simulink model "DriveSystemControl"  (R2023b)
settings: Solver=FixedStepAuto  StartTime=0.0  StopTime=Inf  FixedStep=0.001  RelTol=1e-3
PostLoadFcn:
  | if any(exist('dsrtsu_mdlpostloadfcn', 'file') ~= 0), dsrtsu_mdlpostloadfcn('Execute', bdroot); end
InitFcn:
  | , if any(exist('rtifpga_mdlclblib', 'file') ~= 0), rtifpga_mdlclblib('Init', bdroot); end,
  | , if any(exist('dsmpb_private', 'file') ~= 0), dsmpb_private('dsmpb_mdlclblib', 'Init', bdroot); end,
libraries: dsmpblib x2
(part 7 of 11)

== system DriveSystemControl/Bus Configuration (1) - In/Manipulation/Virya Controller CAN File 08082024/WIP/CANChannel/PDUs/TCU03/sigBPosOvervoltageCutback/Feature Switch ==
  Const_sigBPosOvervoltageCutback Countdown Start Value : Constant  Value=0  OutDataTypeStr=uint32
  Const_sigBPosOvervoltageCutback Feature Switch : Constant  Value=0  OutDataTypeStr=uint32
  _Feature Switch_ : BusCreator  Inputs=2
  Feature Switch : Outport
  wires:
  _Feature Switch_/1 -> Feature Switch/1  "Feature Switch"
  Const_sigBPosOvervoltageCutback Countdown Start Value/1 -> _Feature Switch_/1  "sigBPosOvervoltageCutback Countdown Start Value"
  Const_sigBPosOvervoltageCutback Feature Switch/1 -> _Feature Switch_/2  "sigBPosOvervoltageCutback Feature Switch"

== system DriveSystemControl/Bus Configuration (1) - In/Manipulation/Virya Controller CAN File 08082024/WIP/CANChannel/PDUs/TCU03/sigBPosOvervoltageCutback/ISignal Overwrite Value ==
  Const_sigBPosOvervoltageCutback Overwrite Value : Constant  Value=0  OutDataTypeStr=uint8
  _ISignal Overwrite Value_ : BusCreator  Inputs=1
  ISignal Overwrite Value : Outport
  wires:
  _ISignal Overwrite Value_/1 -> ISignal Overwrite Value/1  "ISignal Overwrite Value"
  Const_sigBPosOvervoltageCutback Overwrite Value/1 -> _ISignal Overwrite Value_/1  "sigBPosOvervoltageCutback Overwrite Value"

== system DriveSystemControl/Bus Configuration (1) - In/Manipulation/Virya Controller CAN File 08082024/WIP/CANChannel/PDUs/TCU03/sigBPosUndervoltageCutback/Feature Switch ==
  Const_sigBPosUndervoltageCutback Countdown Start Value : Constant  Value=0  OutDataTypeStr=uint32
  Const_sigBPosUndervoltageCutback Feature Switch : Constant  Value=0  OutDataTypeStr=uint32
  _Feature Switch_ : BusCreator  Inputs=2
  Feature Switch : Outport
  wires:
  _Feature Switch_/1 -> Feature Switch/1  "Feature Switch"
  Const_sigBPosUndervoltageCutback Countdown Start Value/1 -> _Feature Switch_/1  "sigBPosUndervoltageCutback Countdown Start Value"
  Const_sigBPosUndervoltageCutback Feature Switch/1 -> _Feature Switch_/2  "sigBPosUndervoltageCutback Feature Switch"

== system DriveSystemControl/Bus Configuration (1) - In/Manipulation/Virya Controller CAN File 08082024/WIP/CANChannel/PDUs/TCU03/sigBPosUndervoltageCutback/ISignal Overwrite Value ==
  Const_sigBPosUndervoltageCutback Overwrite Value : Constant  Value=0  OutDataTypeStr=uint8
  _ISignal Overwrite Value_ : BusCreator  Inputs=1
  ISignal Overwrite Value : Outport
  wires:
  _ISignal Overwrite Value_/1 -> ISignal Overwrite Value/1  "ISignal Overwrite Value"
  Const_sigBPosUndervoltageCutback Overwrite Value/1 -> _ISignal Overwrite Value_/1  "sigBPosUndervoltageCutback Overwrite Value"

== system DriveSystemControl/Bus Configuration (1) - In/Manipulation/Virya Controller CAN File 08082024/WIP/CANChannel/PDUs/TCU03/sigBadCalibration/Feature Switch ==
  Const_sigBadCalibration Countdown Start Value : Constant  Value=0  OutDataTypeStr=uint32
  Const_sigBadCalibration Feature Switch : Constant  Value=0  OutDataTypeStr=uint32
  _Feature Switch_ : BusCreator  Inputs=2
  Feature Switch : Outport
  wires:
  _Feature Switch_/1 -> Feature Switch/1  "Feature Switch"
  Const_sigBadCalibration Countdown Start Value/1 -> _Feature Switch_/1  "sigBadCalibration Countdown Start Value"
  Const_sigBadCalibration Feature Switch/1 -> _Feature Switch_/2  "sigBadCalibration Feature Switch"

== system DriveSystemControl/Bus Configuration (1) - In/Manipulation/Virya Controller CAN File 08082024/WIP/CANChannel/PDUs/TCU03/sigBadCalibration/ISignal Overwrite Value ==
  Const_sigBadCalibration Overwrite Value : Constant  Value=0  OutDataTypeStr=uint8
  _ISignal Overwrite Value_ : BusCreator  Inputs=1
  ISignal Overwrite Value : Outport
  wires:
  _ISignal Overwrite Value_/1 -> ISignal Overwrite Value/1  "ISignal Overwrite Value"
  Const_sigBadCalibration Overwrite Value/1 -> _ISignal Overwrite Value_/1  "sigBadCalibration Overwrite Value"

== system DriveSystemControl/Bus Configuration (1) - In/Manipulation/Virya Controller CAN File 08082024/WIP/CANChannel/PDUs/TCU03/sigBrakeWiperHigh/Feature Switch ==
  Const_sigBrakeWiperHigh Countdown Start Value : Constant  Value=0  OutDataTypeStr=uint32
  Const_sigBrakeWiperHigh Feature Switch : Constant  Value=0  OutDataTypeStr=uint32
  _Feature Switch_ : BusCreator  Inputs=2
  Feature Switch : Outport
  wires:
  _Feature Switch_/1 -> Feature Switch/1  "Feature Switch"
  Const_sigBrakeWiperHigh Countdown Start Value/1 -> _Feature Switch_/1  "sigBrakeWiperHigh Countdown Start Value"
  Const_sigBrakeWiperHigh Feature Switch/1 -> _Feature Switch_/2  "sigBrakeWiperHigh Feature Switch"

== system DriveSystemControl/Bus Configuration (1) - In/Manipulation/Virya Controller CAN File 08082024/WIP/CANChannel/PDUs/TCU03/sigBrakeWiperHigh/ISignal Overwrite Value ==
  Const_sigBrakeWiperHigh Overwrite Value : Constant  Value=0  OutDataTypeStr=uint8
  _ISignal Overwrite Value_ : BusCreator  Inputs=1
  ISignal Overwrite Value : Outport
  wires:
  _ISignal Overwrite Value_/1 -> ISignal Overwrite Value/1  "ISignal Overwrite Value"
  Const_sigBrakeWiperHigh Overwrite Value/1 -> _ISignal Overwrite Value_/1  "sigBrakeWiperHigh Overwrite Value"

== system DriveSystemControl/Bus Configuration (1) - In/Manipulation/Virya Controller CAN File 08082024/WIP/CANChannel/PDUs/TCU03/sigBrakeWiperLow/Feature Switch ==
  Const_sigBrakeWiperLow Countdown Start Value : Constant  Value=0  OutDataTypeStr=uint32
  Const_sigBrakeWiperLow Feature Switch : Constant  Value=0  OutDataTypeStr=uint32
  _Feature Switch_ : BusCreator  Inputs=2
  Feature Switch : Outport
  wires:
  _Feature Switch_/1 -> Feature Switch/1  "Feature Switch"
  Const_sigBrakeWiperLow Countdown Start Value/1 -> _Feature Switch_/1  "sigBrakeWiperLow Countdown Start Value"
  Const_sigBrakeWiperLow Feature Switch/1 -> _Feature Switch_/2  "sigBrakeWiperLow Feature Switch"

== system DriveSystemControl/Bus Configuration (1) - In/Manipulation/Virya Controller CAN File 08082024/WIP/CANChannel/PDUs/TCU03/sigBrakeWiperLow/ISignal Overwrite Value ==
  Const_sigBrakeWiperLow Overwrite Value : Constant  Value=0  OutDataTypeStr=uint8
  _ISignal Overwrite Value_ : BusCreator  Inputs=1
  ISignal Overwrite Value : Outport
  wires:
  _ISignal Overwrite Value_/1 -> ISignal Overwrite Value/1  "ISignal Overwrite Value"
  Const_sigBrakeWiperLow Overwrite Value/1 -> _ISignal Overwrite Value_/1  "sigBrakeWiperLow Overwrite Value"

== system DriveSystemControl/Bus Configuration (1) - In/Manipulation/Virya Controller CAN File 08082024/WIP/CANChannel/PDUs/TCU03/sigCoil2DriverOpenShort/Feature Switch ==
  Const_sigCoil2DriverOpenShort Countdown Start Value : Constant  Value=0  OutDataTypeStr=uint32
  Const_sigCoil2DriverOpenShort Feature Switch : Constant  Value=0  OutDataTypeStr=uint32
  _Feature Switch_ : BusCreator  Inputs=2
  Feature Switch : Outport
  wires:
  _Feature Switch_/1 -> Feature Switch/1  "Feature Switch"
  Const_sigCoil2DriverOpenShort Countdown Start Value/1 -> _Feature Switch_/1  "sigCoil2DriverOpenShort Countdown Start Value"
  Const_sigCoil2DriverOpenShort Feature Switch/1 -> _Feature Switch_/2  "sigCoil2DriverOpenShort Feature Switch"

== system DriveSystemControl/Bus Configuration (1) - In/Manipulation/Virya Controller CAN File 08082024/WIP/CANChannel/PDUs/TCU03/sigCoil2DriverOpenShort/ISignal Overwrite Value ==
  Const_sigCoil2DriverOpenShort Overwrite Value : Constant  Value=0  OutDataTypeStr=uint8
  _ISignal Overwrite Value_ : BusCreator  Inputs=1
  ISignal Overwrite Value : Outport
  wires:
  _ISignal Overwrite Value_/1 -> ISignal Overwrite Value/1  "ISignal Overwrite Value"
  Const_sigCoil2DriverOpenShort Overwrite Value/1 -> _ISignal Overwrite Value_/1  "sigCoil2DriverOpenShort Overwrite Value"

== system DriveSystemControl/Bus Configuration (1) - In/Manipulation/Virya Controller CAN File 08082024/WIP/CANChannel/PDUs/TCU03/sigCoil3DriverOpenShort/Feature Switch ==
  Const_sigCoil3DriverOpenShort Countdown Start Value : Constant  Value=0  OutDataTypeStr=uint32
  Const_sigCoil3DriverOpenShort Feature Switch : Constant  Value=0  OutDataTypeStr=uint32
  _Feature Switch_ : BusCreator  Inputs=2
  Feature Switch : Outport
  wires:
  _Feature Switch_/1 -> Feature Switch/1  "Feature Switch"
  Const_sigCoil3DriverOpenShort Countdown Start Value/1 -> _Feature Switch_/1  "sigCoil3DriverOpenShort Countdown Start Value"
  Const_sigCoil3DriverOpenShort Feature Switch/1 -> _Feature Switch_/2  "sigCoil3DriverOpenShort Feature Switch"

== system DriveSystemControl/Bus Configuration (1) - In/Manipulation/Virya Controller CAN File 08082024/WIP/CANChannel/PDUs/TCU03/sigCoil3DriverOpenShort/ISignal Overwrite Value ==
  Const_sigCoil3DriverOpenShort Overwrite Value : Constant  Value=0  OutDataTypeStr=uint8
  _ISignal Overwrite Value_ : BusCreator  Inputs=1
  ISignal Overwrite Value : Outport
  wires:
  _ISignal Overwrite Value_/1 -> ISignal Overwrite Value/1  "ISignal Overwrite Value"
  Const_sigCoil3DriverOpenShort Overwrite Value/1 -> _ISignal Overwrite Value_/1  "sigCoil3DriverOpenShort Overwrite Value"

== system DriveSystemControl/Bus Configuration (1) - In/Manipulation/Virya Controller CAN File 08082024/WIP/CANChannel/PDUs/TCU03/sigCoil4DriverOpenShort/Feature Switch ==
  Const_sigCoil4DriverOpenShort Countdown Start Value : Constant  Value=0  OutDataTypeStr=uint32
  Const_sigCoil4DriverOpenShort Feature Switch : Constant  Value=0  OutDataTypeStr=uint32
  _Feature Switch_ : BusCreator  Inputs=2
  Feature Switch : Outport
  wires:
  _Feature Switch_/1 -> Feature Switch/1  "Feature Switch"
  Const_sigCoil4DriverOpenShort Countdown Start Value/1 -> _Feature Switch_/1  "sigCoil4DriverOpenShort Countdown Start Value"
  Const_sigCoil4DriverOpenShort Feature Switch/1 -> _Feature Switch_/2  "sigCoil4DriverOpenShort Feature Switch"

== system DriveSystemControl/Bus Configuration (1) - In/Manipulation/Virya Controller CAN File 08082024/WIP/CANChannel/PDUs/TCU03/sigCoil4DriverOpenShort/ISignal Overwrite Value ==
  Const_sigCoil4DriverOpenShort Overwrite Value : Constant  Value=0  OutDataTypeStr=uint8
  _ISignal Overwrite Value_ : BusCreator  Inputs=1
  ISignal Overwrite Value : Outport
  wires:
  _ISignal Overwrite Value_/1 -> ISignal Overwrite Value/1  "ISignal Overwrite Value"
  Const_sigCoil4DriverOpenShort Overwrite Value/1 -> _ISignal Overwrite Value_/1  "sigCoil4DriverOpenShort Overwrite Value"

== system DriveSystemControl/Bus Configuration (1) - In/Manipulation/Virya Controller CAN File 08082024/WIP/CANChannel/PDUs/TCU03/sigControllerCommonFault/Feature Switch ==
  Const_sigControllerCommonFault Countdown Start Value : Constant  Value=0  OutDataTypeStr=uint32
  Const_sigControllerCommonFault Feature Switch : Constant  Value=0  OutDataTypeStr=uint32
  _Feature Switch_ : BusCreator  Inputs=2
  Feature Switch : Outport
  wires:
  _Feature Switch_/1 -> Feature Switch/1  "Feature Switch"
  Const_sigControllerCommonFault Countdown Start Value/1 -> _Feature Switch_/1  "sigControllerCommonFault Countdown Start Value"
  Const_sigControllerCommonFault Feature Switch/1 -> _Feature Switch_/2  "sigControllerCommonFault Feature Switch"

== system DriveSystemControl/Bus Configuration (1) - In/Manipulation/Virya Controller CAN File 08082024/WIP/CANChannel/PDUs/TCU03/sigControllerCommonFault/ISignal Overwrite Value ==
  Const_sigControllerCommonFault Overwrite Value : Constant  Value=0  OutDataTypeStr=uint8
  _ISignal Overwrite Value_ : BusCreator  Inputs=1
  ISignal Overwrite Value : Outport
  wires:
  _ISignal Overwrite Value_/1 -> ISignal Overwrite Value/1  "ISignal Overwrite Value"
  Const_sigControllerCommonFault Overwrite Value/1 -> _ISignal Overwrite Value_/1  "sigControllerCommonFault Overwrite Value"

== system DriveSystemControl/Bus Configuration (1) - In/Manipulation/Virya Controller CAN File 08082024/WIP/CANChannel/PDUs/TCU03/sigControllerOverCurrent/Feature Switch ==
  Const_sigControllerOverCurrent Countdown Start Value : Constant  Value=0  OutDataTypeStr=uint32
  Const_sigControllerOverCurrent Feature Switch : Constant  Value=0  OutDataTypeStr=uint32
  _Feature Switch_ : BusCreator  Inputs=2
  Feature Switch : Outport
  wires:
  _Feature Switch_/1 -> Feature Switch/1  "Feature Switch"
  Const_sigControllerOverCurrent Countdown Start Value/1 -> _Feature Switch_/1  "sigControllerOverCurrent Countdown Start Value"
  Const_sigControllerOverCurrent Feature Switch/1 -> _Feature Switch_/2  "sigControllerOverCurrent Feature Switch"

== system DriveSystemControl/Bus Configuration (1) - In/Manipulation/Virya Controller CAN File 08082024/WIP/CANChannel/PDUs/TCU03/sigControllerOverCurrent/ISignal Overwrite Value ==
  Const_sigControllerOverCurrent Overwrite Value : Constant  Value=0  OutDataTypeStr=uint8
  _ISignal Overwrite Value_ : BusCreator  Inputs=1
  ISignal Overwrite Value : Outport
  wires:
  _ISignal Overwrite Value_/1 -> ISignal Overwrite Value/1  "ISignal Overwrite Value"
  Const_sigControllerOverCurrent Overwrite Value/1 -> _ISignal Overwrite Value_/1  "sigControllerOverCurrent Overwrite Value"

== system DriveSystemControl/Bus Configuration (1) - In/Manipulation/Virya Controller CAN File 08082024/WIP/CANChannel/PDUs/TCU03/sigControllerOvertempCutback/Feature Switch ==
  Const_sigControllerOvertempCutback Countdown Start Value : Constant  Value=0  OutDataTypeStr=uint32
  Const_sigControllerOvertempCutback Feature Switch : Constant  Value=0  OutDataTypeStr=uint32
  _Feature Switch_ : BusCreator  Inputs=2
  Feature Switch : Outport
  wires:
  _Feature Switch_/1 -> Feature Switch/1  "Feature Switch"
  Const_sigControllerOvertempCutback Countdown Start Value/1 -> _Feature Switch_/1  "sigControllerOvertempCutback Countdown Start Value"
  Const_sigControllerOvertempCutback Feature Switch/1 -> _Feature Switch_/2  "sigControllerOvertempCutback Feature Switch"

== system DriveSystemControl/Bus Configuration (1) - In/Manipulation/Virya Controller CAN File 08082024/WIP/CANChannel/PDUs/TCU03/sigControllerOvertempCutback/ISignal Overwrite Value ==
  Const_sigControllerOvertempCutback Overwrite Value : Constant  Value=0  OutDataTypeStr=uint8
  _ISignal Overwrite Value_ : BusCreator  Inputs=1
  ISignal Overwrite Value : Outport
  wires:
  _ISignal Overwrite Value_/1 -> ISignal Overwrite Value/1  "ISignal Overwrite Value"
  Const_sigControllerOvertempCutback Overwrite Value/1 -> _ISignal Overwrite Value_/1  "sigControllerOvertempCutback Overwrite Value"

== system DriveSystemControl/Bus Configuration (1) - In/Manipulation/Virya Controller CAN File 08082024/WIP/CANChannel/PDUs/TCU03/sigControllerSevereOvertemp/Feature Switch ==
  Const_sigControllerSevereOvertemp Countdown Start Value : Constant  Value=0  OutDataTypeStr=uint32
  Const_sigControllerSevereOvertemp Feature Switch : Constant  Value=0  OutDataTypeStr=uint32
  _Feature Switch_ : BusCreator  Inputs=2
  Feature Switch : Outport
  wires:
  _Feature Switch_/1 -> Feature Switch/1  "Feature Switch"
  Const_sigControllerSevereOvertemp Countdown Start Value/1 -> _Feature Switch_/1  "sigControllerSevereOvertemp Countdown Start Value"
  Const_sigControllerSevereOvertemp Feature Switch/1 -> _Feature Switch_/2  "sigControllerSevereOvertemp Feature Switch"

== system DriveSystemControl/Bus Configuration (1) - In/Manipulation/Virya Controller CAN File 08082024/WIP/CANChannel/PDUs/TCU03/sigControllerSevereOvertemp/ISignal Overwrite Value ==
  Const_sigControllerSevereOvertemp Overwrite Value : Constant  Value=0  OutDataTypeStr=uint8
  _ISignal Overwrite Value_ : BusCreator  Inputs=1
  ISignal Overwrite Value : Outport
  wires:
  _ISignal Overwrite Value_/1 -> ISignal Overwrite Value/1  "ISignal Overwrite Value"
  Const_sigControllerSevereOvertemp Overwrite Value/1 -> _ISignal Overwrite Value_/1  "sigControllerSevereOvertemp Overwrite Value"

== system DriveSystemControl/Bus Configuration (1) - In/Manipulation/Virya Controller CAN File 08082024/WIP/CANChannel/PDUs/TCU03/sigControllerSevereUndertemp/Feature Switch ==
  Const_sigControllerSevereUndertemp Countdown Start Value : Constant  Value=0  OutDataTypeStr=uint32
  Const_sigControllerSevereUndertemp Feature Switch : Constant  Value=0  OutDataTypeStr=uint32
  _Feature Switch_ : BusCreator  Inputs=2
  Feature Switch : Outport
  wires:
  _Feature Switch_/1 -> Feature Switch/1  "Feature Switch"
  Const_sigControllerSevereUndertemp Countdown Start Value/1 -> _Feature Switch_/1  "sigControllerSevereUndertemp Countdown Start Value"
  Const_sigControllerSevereUndertemp Feature Switch/1 -> _Feature Switch_/2  "sigControllerSevereUndertemp Feature Switch"

== system DriveSystemControl/Bus Configuration (1) - In/Manipulation/Virya Controller CAN File 08082024/WIP/CANChannel/PDUs/TCU03/sigControllerSevereUndertemp/ISignal Overwrite Value ==
  Const_sigControllerSevereUndertemp Overwrite Value : Constant  Value=0  OutDataTypeStr=uint8
  _ISignal Overwrite Value_ : BusCreator  Inputs=1
  ISignal Overwrite Value : Outport
  wires:
  _ISignal Overwrite Value_/1 -> ISignal Overwrite Value/1  "ISignal Overwrite Value"
  Const_sigControllerSevereUndertemp Overwrite Value/1 -> _ISignal Overwrite Value_/1  "sigControllerSevereUndertemp Overwrite Value"

== system DriveSystemControl/Bus Configuration (1) - In/Manipulation/Virya Controller CAN File 08082024/WIP/CANChannel/PDUs/TCU03/sigCurrentSensorFault/Feature Switch ==
  Const_sigCurrentSensorFault Countdown Start Value : Constant  Value=0  OutDataTypeStr=uint32
  Const_sigCurrentSensorFault Feature Switch : Constant  Value=0  OutDataTypeStr=uint32
  _Feature Switch_ : BusCreator  Inputs=2
  Feature Switch : Outport
  wires:
  _Feature Switch_/1 -> Feature Switch/1  "Feature Switch"
  Const_sigCurrentSensorFault Countdown Start Value/1 -> _Feature Switch_/1  "sigCurrentSensorFault Countdown Start Value"
  Const_sigCurrentSensorFault Feature Switch/1 -> _Feature Switch_/2  "sigCurrentSensorFault Feature Switch"

== system DriveSystemControl/Bus Configuration (1) - In/Manipulation/Virya Controller CAN File 08082024/WIP/CANChannel/PDUs/TCU03/sigCurrentSensorFault/ISignal Overwrite Value ==
  Const_sigCurrentSensorFault Overwrite Value : Constant  Value=0  OutDataTypeStr=uint8
  _ISignal Overwrite Value_ : BusCreator  Inputs=1
  ISignal Overwrite Value : Outport
  wires:
  _ISignal Overwrite Value_/1 -> ISignal Overwrite Value/1  "ISignal Overwrite Value"
  Const_sigCurrentSensorFault Overwrite Value/1 -> _ISignal Overwrite Value_/1  "sigCurrentSensorFault Overwrite Value"

== system DriveSystemControl/Bus Configuration (1) - In/Manipulation/Virya Controller CAN File 08082024/WIP/CANChannel/PDUs/TCU03/sigEEPROMFailure/Feature Switch ==
  Const_sigEEPROMFailure Countdown Start Value : Constant  Value=0  OutDataTypeStr=uint32
  Const_sigEEPROMFailure Feature Switch : Constant  Value=0  OutDataTypeStr=uint32
  _Feature Switch_ : BusCreator  Inputs=2
  Feature Switch : Outport
  wires:
  _Feature Switch_/1 -> Feature Switch/1  "Feature Switch"
  Const_sigEEPROMFailure Countdown Start Value/1 -> _Feature Switch_/1  "sigEEPROMFailure Countdown Start Value"
  Const_sigEEPROMFailure Feature Switch/1 -> _Feature Switch_/2  "sigEEPROMFailure Feature Switch"

== system DriveSystemControl/Bus Configuration (1) - In/Manipulation/Virya Controller CAN File 08082024/WIP/CANChannel/PDUs/TCU03/sigEEPROMFailure/ISignal Overwrite Value ==
  Const_sigEEPROMFailure Overwrite Value : Constant  Value=0  OutDataTypeStr=uint8
  _ISignal Overwrite Value_ : BusCreator  Inputs=1
  ISignal Overwrite Value : Outport
  wires:
  _ISignal Overwrite Value_/1 -> ISignal Overwrite Value/1  "ISignal Overwrite Value"
  Const_sigEEPROMFailure Overwrite Value/1 -> _ISignal Overwrite Value_/1  "sigEEPROMFailure Overwrite Value"

== system DriveSystemControl/Bus Configuration (1) - In/Manipulation/Virya Controller CAN File 08082024/WIP/CANChannel/PDUs/TCU03/sigHighPedalDisable/Feature Switch ==
  Const_sigHighPedalDisable Countdown Start Value : Constant  Value=0  OutDataTypeStr=uint32
  Const_sigHighPedalDisable Feature Switch : Constant  Value=0  OutDataTypeStr=uint32
  _Feature Switch_ : BusCreator  Inputs=2
  Feature Switch : Outport
  wires:
  _Feature Switch_/1 -> Feature Switch/1  "Feature Switch"
  Const_sigHighPedalDisable Countdown Start Value/1 -> _Feature Switch_/1  "sigHighPedalDisable Countdown Start Value"
  Const_sigHighPedalDisable Feature Switch/1 -> _Feature Switch_/2  "sigHighPedalDisable Feature Switch"

== system DriveSystemControl/Bus Configuration (1) - In/Manipulation/Virya Controller CAN File 08082024/WIP/CANChannel/PDUs/TCU03/sigHighPedalDisable/ISignal Overwrite Value ==
  Const_sigHighPedalDisable Overwrite Value : Constant  Value=0  OutDataTypeStr=uint8
  _ISignal Overwrite Value_ : BusCreator  Inputs=1
  ISignal Overwrite Value : Outport
  wires:
  _ISignal Overwrite Value_/1 -> ISignal Overwrite Value/1  "ISignal Overwrite Value"
  Const_sigHighPedalDisable Overwrite Value/1 -> _ISignal Overwrite Value_/1  "sigHighPedalDisable Overwrite Value"

== system DriveSystemControl/Bus Configuration (1) - In/Manipulation/Virya Controller CAN File 08082024/WIP/CANChannel/PDUs/TCU03/sigInsulationResistanceLow/Feature Switch ==
  Const_sigInsulationResistanceLow Countdown Start Value : Constant  Value=0  OutDataTypeStr=uint32
  Const_sigInsulationResistanceLow Feature Switch : Constant  Value=0  OutDataTypeStr=uint32
  _Feature Switch_ : BusCreator  Inputs=2
  Feature Switch : Outport
  wires:
  _Feature Switch_/1 -> Feature Switch/1  "Feature Switch"
  Const_sigInsulationResistanceLow Countdown Start Value/1 -> _Feature Switch_/1  "sigInsulationResistanceLow Countdown Start Value"
  Const_sigInsulationResistanceLow Feature Switch/1 -> _Feature Switch_/2  "sigInsulationResistanceLow Feature Switch"

== system DriveSystemControl/Bus Configuration (1) - In/Manipulation/Virya Controller CAN File 08082024/WIP/CANChannel/PDUs/TCU03/sigInsulationResistanceLow/ISignal Overwrite Value ==
  Const_sigInsulationResistanceLow Overwrite Value : Constant  Value=0  OutDataTypeStr=uint8
  _ISignal Overwrite Value_ : BusCreator  Inputs=1
  ISignal Overwrite Value : Outport
  wires:
  _ISignal Overwrite Value_/1 -> ISignal Overwrite Value/1  "ISignal Overwrite Value"
  Const_sigInsulationResistanceLow Overwrite Value/1 -> _ISignal Overwrite Value_/1  "sigInsulationResistanceLow Overwrite Value"

== system DriveSystemControl/Bus Configuration (1) - In/Manipulation/Virya Controller CAN File 08082024/WIP/CANChannel/PDUs/TCU03/sigMainContactorWelded/Feature Switch ==
  Const_sigMainContactorWelded Countdown Start Value : Constant  Value=0  OutDataTypeStr=uint32
  Const_sigMainContactorWelded Feature Switch : Constant  Value=0  OutDataTypeStr=uint32
  _Feature Switch_ : BusCreator  Inputs=2
  Feature Switch : Outport
  wires:
  _Feature Switch_/1 -> Feature Switch/1  "Feature Switch"
  Const_sigMainContactorWelded Countdown Start Value/1 -> _Feature Switch_/1  "sigMainContactorWelded Countdown Start Value"
  Const_sigMainContactorWelded Feature Switch/1 -> _Feature Switch_/2  "sigMainContactorWelded Feature Switch"

== system DriveSystemControl/Bus Configuration (1) - In/Manipulation/Virya Controller CAN File 08082024/WIP/CANChannel/PDUs/TCU03/sigMainContactorWelded/ISignal Overwrite Value ==
  Const_sigMainContactorWelded Overwrite Value : Constant  Value=0  OutDataTypeStr=uint8
  _ISignal Overwrite Value_ : BusCreator  Inputs=1
  ISignal Overwrite Value : Outport
  wires:
  _ISignal Overwrite Value_/1 -> ISignal Overwrite Value/1  "ISignal Overwrite Value"
  Const_sigMainContactorWelded Overwrite Value/1 -> _ISignal Overwrite Value_/1  "sigMainContactorWelded Overwrite Value"

== system DriveSystemControl/Bus Configuration (1) - In/Manipulation/Virya Controller CAN File 08082024/WIP/CANChannel/PDUs/TCU03/sigMainContactordidnotClose/Feature Switch ==
  Const_sigMainContactordidnotClose Countdown Start Value : Constant  Value=0  OutDataTypeStr=uint32
  Const_sigMainContactordidnotClose Feature Switch : Constant  Value=0  OutDataTypeStr=uint32
  _Feature Switch_ : BusCreator  Inputs=2
  Feature Switch : Outport
  wires:
  _Feature Switch_/1 -> Feature Switch/1  "Feature Switch"
  Const_sigMainContactordidnotClose Countdown Start Value/1 -> _Feature Switch_/1  "sigMainContactordidnotClose Countdown Start Value"
  Const_sigMainContactordidnotClose Feature Switch/1 -> _Feature Switch_/2  "sigMainContactordidnotClose Feature Switch"

== system DriveSystemControl/Bus Configuration (1) - In/Manipulation/Virya Controller CAN File 08082024/WIP/CANChannel/PDUs/TCU03/sigMainContactordidnotClose/ISignal Overwrite Value ==
  Const_sigMainContactordidnotClose Overwrite Value : Constant  Value=0  OutDataTypeStr=uint8
  _ISignal Overwrite Value_ : BusCreator  Inputs=1
  ISignal Overwrite Value : Outport
  wires:
  _ISignal Overwrite Value_/1 -> ISignal Overwrite Value/1  "ISignal Overwrite Value"
  Const_sigMainContactordidnotClose Overwrite Value/1 -> _ISignal Overwrite Value_/1  "sigMainContactordidnotClose Overwrite Value"

== system DriveSystemControl/Bus Configuration (1) - In/Manipulation/Virya Controller CAN File 08082024/WIP/CANChannel/PDUs/TCU03/sigMainOpenShort/Feature Switch ==
  Const_sigMainOpenShort Countdown Start Value : Constant  Value=0  OutDataTypeStr=uint32
  Const_sigMainOpenShort Feature Switch : Constant  Value=0  OutDataTypeStr=uint32
  _Feature Switch_ : BusCreator  Inputs=2
  Feature Switch : Outport
  wires:
  _Feature Switch_/1 -> Feature Switch/1  "Feature Switch"
  Const_sigMainOpenShort Countdown Start Value/1 -> _Feature Switch_/1  "sigMainOpenShort Countdown Start Value"
  Const_sigMainOpenShort Feature Switch/1 -> _Feature Switch_/2  "sigMainOpenShort Feature Switch"

== system DriveSystemControl/Bus Configuration (1) - In/Manipulation/Virya Controller CAN File 08082024/WIP/CANChannel/PDUs/TCU03/sigMainOpenShort/ISignal Overwrite Value ==
  Const_sigMainOpenShort Overwrite Value : Constant  Value=0  OutDataTypeStr=uint8
  _ISignal Overwrite Value_ : BusCreator  Inputs=1
  ISignal Overwrite Value : Outport
  wires:
  _ISignal Overwrite Value_/1 -> ISignal Overwrite Value/1  "ISignal Overwrite Value"
  Const_sigMainOpenShort Overwrite Value/1 -> _ISignal Overwrite Value_/1  "sigMainOpenShort Overwrite Value"

== system DriveSystemControl/Bus Configuration (1) - In/Manipulation/Virya Controller CAN File 08082024/WIP/CANChannel/PDUs/TCU03/sigMotorCharacterization/Feature Switch ==
  Const_sigMotorCharacterization Countdown Start Value : Constant  Value=0  OutDataTypeStr=uint32
  Const_sigMotorCharacterization Feature Switch : Constant  Value=0  OutDataTypeStr=uint32
  _Feature Switch_ : BusCreator  Inputs=2
  Feature Switch : Outport
  wires:
  _Feature Switch_/1 -> Feature Switch/1  "Feature Switch"
  Const_sigMotorCharacterization Countdown Start Value/1 -> _Feature Switch_/1  "sigMotorCharacterization Countdown Start Value"
  Const_sigMotorCharacterization Feature Switch/1 -> _Feature Switch_/2  "sigMotorCharacterization Feature Switch"

== system DriveSystemControl/Bus Configuration (1) - In/Manipulation/Virya Controller CAN File 08082024/WIP/CANChannel/PDUs/TCU03/sigMotorCharacterization/ISignal Overwrite Value ==
  Const_sigMotorCharacterization Overwrite Value : Constant  Value=0  OutDataTypeStr=uint8
  _ISignal Overwrite Value_ : BusCreator  Inputs=1
  ISignal Overwrite Value : Outport
  wires:
  _ISignal Overwrite Value_/1 -> ISignal Overwrite Value/1  "ISignal Overwrite Value"
  Const_sigMotorCharacterization Overwrite Value/1 -> _ISignal Overwrite Value_/1  "sigMotorCharacterization Overwrite Value"

== system DriveSystemControl/Bus Configuration (1) - In/Manipulation/Virya Controller CAN File 08082024/WIP/CANChannel/PDUs/TCU03/sigMotorPhaseOpen/Feature Switch ==
  Const_sigMotorPhaseOpen Countdown Start Value : Constant  Value=0  OutDataTypeStr=uint32
  Const_sigMotorPhaseOpen Feature Switch : Constant  Value=0  OutDataTypeStr=uint32
  _Feature Switch_ : BusCreator  Inputs=2
  Feature Switch : Outport
  wires:
  _Feature Switch_/1 -> Feature Switch/1  "Feature Switch"
  Const_sigMotorPhaseOpen Countdown Start Value/1 -> _Feature Switch_/1  "sigMotorPhaseOpen Countdown Start Value"
  Const_sigMotorPhaseOpen Feature Switch/1 -> _Feature Switch_/2  "sigMotorPhaseOpen Feature Switch"

== system DriveSystemControl/Bus Configuration (1) - In/Manipulation/Virya Controller CAN File 08082024/WIP/CANChannel/PDUs/TCU03/sigMotorPhaseOpen/ISignal Overwrite Value ==
  Const_sigMotorPhaseOpen Overwrite Value : Constant  Value=0  OutDataTypeStr=uint8
  _ISignal Overwrite Value_ : BusCreator  Inputs=1
  ISignal Overwrite Value : Outport
  wires:
  _ISignal Overwrite Value_/1 -> ISignal Overwrite Value/1  "ISignal Overwrite Value"
  Const_sigMotorPhaseOpen Overwrite Value/1 -> _ISignal Overwrite Value_/1  "sigMotorPhaseOpen Overwrite Value"

== system DriveSystemControl/Bus Configuration (1) - In/Manipulation/Virya Controller CAN File 08082024/WIP/CANChannel/PDUs/TCU03/sigMotorTempHotCutback/Feature Switch ==
  Const_sigMotorTempHotCutback Countdown Start Value : Constant  Value=0  OutDataTypeStr=uint32
  Const_sigMotorTempHotCutback Feature Switch : Constant  Value=0  OutDataTypeStr=uint32
  _Feature Switch_ : BusCreator  Inputs=2
  Feature Switch : Outport
  wires:
  _Feature Switch_/1 -> Feature Switch/1  "Feature Switch"
  Const_sigMotorTempHotCutback Countdown Start Value/1 -> _Feature Switch_/1  "sigMotorTempHotCutback Countdown Start Value"
  Const_sigMotorTempHotCutback Feature Switch/1 -> _Feature Switch_/2  "sigMotorTempHotCutback Feature Switch"

== system DriveSystemControl/Bus Configuration (1) - In/Manipulation/Virya Controller CAN File 08082024/WIP/CANChannel/PDUs/TCU03/sigMotorTempHotCutback/ISignal Overwrite Value ==
  Const_sigMotorTempHotCutback Overwrite Value : Constant  Value=0  OutDataTypeStr=uint8
  _ISignal Overwrite Value_ : BusCreator  Inputs=1
  ISignal Overwrite Value : Outport
  wires:
  _ISignal Overwrite Value_/1 -> ISignal Overwrite Value/1  "ISignal Overwrite Value"
  Const_sigMotorTempHotCutback Overwrite Value/1 -> _ISignal Overwrite Value_/1  "sigMotorTempHotCutback Overwrite Value"

== system DriveSystemControl/Bus Configuration (1) - In/Manipulation/Virya Controller CAN File 08082024/WIP/CANChannel/PDUs/TCU03/sigMotorTempSensorFault/Feature Switch ==
  Const_sigMotorTempSensorFault Countdown Start Value : Constant  Value=0  OutDataTypeStr=uint32
  Const_sigMotorTempSensorFault Feature Switch : Constant  Value=0  OutDataTypeStr=uint32
  _Feature Switch_ : BusCreator  Inputs=2
  Feature Switch : Outport
  wires:
  _Feature Switch_/1 -> Feature Switch/1  "Feature Switch"
  Const_sigMotorTempSensorFault Countdown Start Value/1 -> _Feature Switch_/1  "sigMotorTempSensorFault Countdown Start Value"
  Const_sigMotorTempSensorFault Feature Switch/1 -> _Feature Switch_/2  "sigMotorTempSensorFault Feature Switch"

== system DriveSystemControl/Bus Configuration (1) - In/Manipulation/Virya Controller CAN File 08082024/WIP/CANChannel/PDUs/TCU03/sigMotorTempSensorFault/ISignal Overwrite Value ==
  Const_sigMotorTempSensorFault Overwrite Value : Constant  Value=0  OutDataTypeStr=uint8
  _ISignal Overwrite Value_ : BusCreator  Inputs=1
  ISignal Overwrite Value : Outport
  wires:
  _ISignal Overwrite Value_/1 -> ISignal Overwrite Value/1  "ISignal Overwrite Value"
  Const_sigMotorTempSensorFault Overwrite Value/1 -> _ISignal Overwrite Value_/1  "sigMotorTempSensorFault Overwrite Value"

== system DriveSystemControl/Bus Configuration (1) - In/Manipulation/Virya Controller CAN File 08082024/WIP/CANChannel/PDUs/TCU03/sigOEM_BatterySTOPSignal/Feature Switch ==
  Const_sigOEM_BatterySTOPSignal Countdown Start Value : Constant  Value=0  OutDataTypeStr=uint32
  Const_sigOEM_BatterySTOPSignal Feature Switch : Constant  Value=0  OutDataTypeStr=uint32
  _Feature Switch_ : BusCreator  Inputs=2
  Feature Switch : Outport
  wires:
  _Feature Switch_/1 -> Feature Switch/1  "Feature Switch"
  Const_sigOEM_BatterySTOPSignal Countdown Start Value/1 -> _Feature Switch_/1  "sigOEM_BatterySTOPSignal Countdown Start Value"
  Const_sigOEM_BatterySTOPSignal Feature Switch/1 -> _Feature Switch_/2  "sigOEM_BatterySTOPSignal Feature Switch"

== system DriveSystemControl/Bus Configuration (1) - In/Manipulation/Virya Controller CAN File 08082024/WIP/CANChannel/PDUs/TCU03/sigOEM_BatterySTOPSignal/ISignal Overwrite Value ==
  Const_sigOEM_BatterySTOPSignal Overwrite Value : Constant  Value=0  OutDataTypeStr=uint8
  _ISignal Overwrite Value_ : BusCreator  Inputs=1
  ISignal Overwrite Value : Outport
  wires:
  _ISignal Overwrite Value_/1 -> ISignal Overwrite Value/1  "ISignal Overwrite Value"
  Const_sigOEM_BatterySTOPSignal Overwrite Value/1 -> _ISignal Overwrite Value_/1  "sigOEM_BatterySTOPSignal Overwrite Value"

== system DriveSystemControl/Bus Configuration (1) - In/Manipulation/Virya Controller CAN File 08082024/WIP/CANChannel/PDUs/TCU03/sigOEM_NoBatteryCAN/Feature Switch ==
  Const_sigOEM_NoBatteryCAN Countdown Start Value : Constant  Value=0  OutDataTypeStr=uint32
  Const_sigOEM_NoBatteryCAN Feature Switch : Constant  Value=0  OutDataTypeStr=uint32
  _Feature Switch_ : BusCreator  Inputs=2
  Feature Switch : Outport
  wires:
  _Feature Switch_/1 -> Feature Switch/1  "Feature Switch"
  Const_sigOEM_NoBatteryCAN Countdown Start Value/1 -> _Feature Switch_/1  "sigOEM_NoBatteryCAN Countdown Start Value"
  Const_sigOEM_NoBatteryCAN Feature Switch/1 -> _Feature Switch_/2  "sigOEM_NoBatteryCAN Feature Switch"

== system DriveSystemControl/Bus Configuration (1) - In/Manipulation/Virya Controller CAN File 08082024/WIP/CANChannel/PDUs/TCU03/sigOEM_NoBatteryCAN/ISignal Overwrite Value ==
  Const_sigOEM_NoBatteryCAN Overwrite Value : Constant  Value=0  OutDataTypeStr=uint8
  _ISignal Overwrite Value_ : BusCreator  Inputs=1
  ISignal Overwrite Value : Outport
  wires:
  _ISignal Overwrite Value_/1 -> ISignal Overwrite Value/1  "ISignal Overwrite Value"
  Const_sigOEM_NoBatteryCAN Overwrite Value/1 -> _ISignal Overwrite Value_/1  "sigOEM_NoBatteryCAN Overwrite Value"

== system DriveSystemControl/Bus Configuration (1) - In/Manipulation/Virya Controller CAN File 08082024/WIP/CANChannel/PDUs/TCU03/sigOSGeneral/Feature Switch ==
  Const_sigOSGeneral Countdown Start Value : Constant  Value=0  OutDataTypeStr=uint32
  Const_sigOSGeneral Feature Switch : Constant  Value=0  OutDataTypeStr=uint32
  _Feature Switch_ : BusCreator  Inputs=2
  Feature Switch : Outport
  wires:
  _Feature Switch_/1 -> Feature Switch/1  "Feature Switch"
  Const_sigOSGeneral Countdown Start Value/1 -> _Feature Switch_/1  "sigOSGeneral Countdown Start Value"
  Const_sigOSGeneral Feature Switch/1 -> _Feature Switch_/2  "sigOSGeneral Feature Switch"

== system DriveSystemControl/Bus Configuration (1) - In/Manipulation/Virya Controller CAN File 08082024/WIP/CANChannel/PDUs/TCU03/sigOSGeneral/ISignal Overwrite Value ==
  Const_sigOSGeneral Overwrite Value : Constant  Value=0  OutDataTypeStr=uint8
  _ISignal Overwrite Value_ : BusCreator  Inputs=1
  ISignal Overwrite Value : Outport
  wires:
  _ISignal Overwrite Value_/1 -> ISignal Overwrite Value/1  "ISignal Overwrite Value"
  Const_sigOSGeneral Overwrite Value/1 -> _ISignal Overwrite Value_/1  "sigOSGeneral Overwrite Value"

== system DriveSystemControl/Bus Configuration (1) - In/Manipulation/Virya Controller CAN File 08082024/WIP/CANChannel/PDUs/TCU03/sigPMACCommissioningNeeded/Feature Switch ==
  Const_sigPMACCommissioningNeeded Countdown Start Value : Constant  Value=0  OutDataTypeStr=uint32
  Const_sigPMACCommissioningNeeded Feature Switch : Constant  Value=0  OutDataTypeStr=uint32
  _Feature Switch_ : BusCreator  Inputs=2
  Feature Switch : Outport
  wires:
  _Feature Switch_/1 -> Feature Switch/1  "Feature Switch"
  Const_sigPMACCommissioningNeeded Countdown Start Value/1 -> _Feature Switch_/1  "sigPMACCommissioningNeeded Countdown Start Value"
  Const_sigPMACCommissioningNeeded Feature Switch/1 -> _Feature Switch_/2  "sigPMACCommissioningNeeded Feature Switch"

== system DriveSystemControl/Bus Configuration (1) - In/Manipulation/Virya Controller CAN File 08082024/WIP/CANChannel/PDUs/TCU03/sigPMACCommissioningNeeded/ISignal Overwrite Value ==
  Const_sigPMACCommissioningNeeded Overwrite Value : Constant  Value=0  OutDataTypeStr=uint8
  _ISignal Overwrite Value_ : BusCreator  Inputs=1
  ISignal Overwrite Value : Outport
  wires:
  _ISignal Overwrite Value_/1 -> ISignal Overwrite Value/1  "ISignal Overwrite Value"
  Const_sigPMACCommissioningNeeded Overwrite Value/1 -> _ISignal Overwrite Value_/1  "sigPMACCommissioningNeeded Overwrite Value"

== system DriveSystemControl/Bus Configuration (1) - In/Manipulation/Virya Controller CAN File 08082024/WIP/CANChannel/PDUs/TCU03/sigParameterChangeFault/Feature Switch ==
  Const_sigParameterChangeFault Countdown Start Value : Constant  Value=0  OutDataTypeStr=uint32
  Const_sigParameterChangeFault Feature Switch : Constant  Value=0  OutDataTypeStr=uint32
  _Feature Switch_ : BusCreator  Inputs=2
  Feature Switch : Outport
  wires:
  _Feature Switch_/1 -> Feature Switch/1  "Feature Switch"
  Const_sigParameterChangeFault Countdown Start Value/1 -> _Feature Switch_/1  "sigParameterChangeFault Countdown Start Value"
  Const_sigParameterChangeFault Feature Switch/1 -> _Feature Switch_/2  "sigParameterChangeFault Feature Switch"

== system DriveSystemControl/Bus Configuration (1) - In/Manipulation/Virya Controller CAN File 08082024/WIP/CANChannel/PDUs/TCU03/sigParameterChangeFault/ISignal Overwrite Value ==
  Const_sigParameterChangeFault Overwrite Value : Constant  Value=0  OutDataTypeStr=uint8
  _ISignal Overwrite Value_ : BusCreator  Inputs=1
  ISignal Overwrite Value : Outport
  wires:
  _ISignal Overwrite Value_/1 -> ISignal Overwrite Value/1  "ISignal Overwrite Value"
  Const_sigParameterChangeFault Overwrite Value/1 -> _ISignal Overwrite Value_/1  "sigParameterChangeFault Overwrite Value"

== system DriveSystemControl/Bus Configuration (1) - In/Manipulation/Virya Controller CAN File 08082024/WIP/CANChannel/PDUs/TCU03/sigPhasePWMMismatch/Feature Switch ==
  Const_sigPhasePWMMismatch Countdown Start Value : Constant  Value=0  OutDataTypeStr=uint32
  Const_sigPhasePWMMismatch Feature Switch : Constant  Value=0  OutDataTypeStr=uint32
  _Feature Switch_ : BusCreator  Inputs=2
  Feature Switch : Outport
  wires:
  _Feature Switch_/1 -> Feature Switch/1  "Feature Switch"
  Const_sigPhasePWMMismatch Countdown Start Value/1 -> _Feature Switch_/1  "sigPhasePWMMismatch Countdown Start Value"
  Const_sigPhasePWMMismatch Feature Switch/1 -> _Feature Switch_/2  "sigPhasePWMMismatch Feature Switch"

== system DriveSystemControl/Bus Configuration (1) - In/Manipulation/Virya Controller CAN File 08082024/WIP/CANChannel/PDUs/TCU03/sigPhasePWMMismatch/ISignal Overwrite Value ==
  Const_sigPhasePWMMismatch Overwrite Value : Constant  Value=0  OutDataTypeStr=uint8
  _ISignal Overwrite Value_ : BusCreator  Inputs=1
  ISignal Overwrite Value : Outport
  wires:
  _ISignal Overwrite Value_/1 -> ISignal Overwrite Value/1  "ISignal Overwrite Value"
  Const_sigPhasePWMMismatch Overwrite Value/1 -> _ISignal Overwrite Value_/1  "sigPhasePWMMismatch Overwrite Value"

== system DriveSystemControl/Bus Configuration (1) - In/Manipulation/Virya Controller CAN File 08082024/WIP/CANChannel/PDUs/TCU03/sigPrechargeFailed/Feature Switch ==
  Const_sigPrechargeFailed Countdown Start Value : Constant  Value=0  OutDataTypeStr=uint32
  Const_sigPrechargeFailed Feature Switch : Constant  Value=0  OutDataTypeStr=uint32
  _Feature Switch_ : BusCreator  Inputs=2
  Feature Switch : Outport
  wires:
  _Feature Switch_/1 -> Feature Switch/1  "Feature Switch"
  Const_sigPrechargeFailed Countdown Start Value/1 -> _Feature Switch_/1  "sigPrechargeFailed Countdown Start Value"
  Const_sigPrechargeFailed Feature Switch/1 -> _Feature Switch_/2  "sigPrechargeFailed Feature Switch"

== system DriveSystemControl/Bus Configuration (1) - In/Manipulation/Virya Controller CAN File 08082024/WIP/CANChannel/PDUs/TCU03/sigPrechargeFailed/ISignal Overwrite Value ==
  Const_sigPrechargeFailed Overwrite Value : Constant  Value=0  OutDataTypeStr=uint8
  _ISignal Overwrite Value_ : BusCreator  Inputs=1
  ISignal Overwrite Value : Outport
  wires:
  _ISignal Overwrite Value_/1 -> ISignal Overwrite Value/1  "ISignal Overwrite Value"
  Const_sigPrechargeFailed Overwrite Value/1 -> _ISignal Overwrite Value_/1  "sigPrechargeFailed Overwrite Value"

== system DriveSystemControl/Bus Configuration (1) - In/Manipulation/Virya Controller CAN File 08082024/WIP/CANChannel/PDUs/TCU03/sigSevereBPosOvervoltage/Feature Switch ==
  Const_sigSevereBPosOvervoltage Countdown Start Value : Constant  Value=0  OutDataTypeStr=uint32
  Const_sigSevereBPosOvervoltage Feature Switch : Constant  Value=0  OutDataTypeStr=uint32
  _Feature Switch_ : BusCreator  Inputs=2
  Feature Switch : Outport
  wires:
  _Feature Switch_/1 -> Feature Switch/1  "Feature Switch"
  Const_sigSevereBPosOvervoltage Countdown Start Value/1 -> _Feature Switch_/1  "sigSevereBPosOvervoltage Countdown Start Value"
  Const_sigSevereBPosOvervoltage Feature Switch/1 -> _Feature Switch_/2  "sigSevereBPosOvervoltage Feature Switch"

== system DriveSystemControl/Bus Configuration (1) - In/Manipulation/Virya Controller CAN File 08082024/WIP/CANChannel/PDUs/TCU03/sigSevereBPosOvervoltage/ISignal Overwrite Value ==
  Const_sigSevereBPosOvervoltage Overwrite Value : Constant  Value=0  OutDataTypeStr=uint8
  _ISignal Overwrite Value_ : BusCreator  Inputs=1
  ISignal Overwrite Value : Outport
  wires:
  _ISignal Overwrite Value_/1 -> ISignal Overwrite Value/1  "ISignal Overwrite Value"
  Const_sigSevereBPosOvervoltage Overwrite Value/1 -> _ISignal Overwrite Value_/1  "sigSevereBPosOvervoltage Overwrite Value"

== system DriveSystemControl/Bus Configuration (1) - In/Manipulation/Virya Controller CAN File 08082024/WIP/CANChannel/PDUs/TCU03/sigSevereBPosUndervoltage/Feature Switch ==
  Const_sigSevereBPosUndervoltage Countdown Start Value : Constant  Value=0  OutDataTypeStr=uint32
  Const_sigSevereBPosUndervoltage Feature Switch : Constant  Value=0  OutDataTypeStr=uint32
  _Feature Switch_ : BusCreator  Inputs=2
  Feature Switch : Outport
  wires:
  _Feature Switch_/1 -> Feature Switch/1  "Feature Switch"
  Const_sigSevereBPosUndervoltage Countdown Start Value/1 -> _Feature Switch_/1  "sigSevereBPosUndervoltage Countdown Start Value"
  Const_sigSevereBPosUndervoltage Feature Switch/1 -> _Feature Switch_/2  "sigSevereBPosUndervoltage Feature Switch"

== system DriveSystemControl/Bus Configuration (1) - In/Manipulation/Virya Controller CAN File 08082024/WIP/CANChannel/PDUs/TCU03/sigSevereBPosUndervoltage/ISignal Overwrite Value ==
  Const_sigSevereBPosUndervoltage Overwrite Value : Constant  Value=0  OutDataTypeStr=uint8
  _ISignal Overwrite Value_ : BusCreator  Inputs=1
  ISignal Overwrite Value : Outport
  wires:
  _ISignal Overwrite Value_/1 -> ISignal Overwrite Value/1  "ISignal Overwrite Value"
  Const_sigSevereBPosUndervoltage Overwrite Value/1 -> _ISignal Overwrite Value_/1  "sigSevereBPosUndervoltage Overwrite Value"

== system DriveSystemControl/Bus Configuration (1) - In/Manipulation/Virya Controller CAN File 08082024/WIP/CANChannel/PDUs/TCU03/sigSevereKSIOvervoltage/Feature Switch ==
  Const_sigSevereKSIOvervoltage Countdown Start Value : Constant  Value=0  OutDataTypeStr=uint32
  Const_sigSevereKSIOvervoltage Feature Switch : Constant  Value=0  OutDataTypeStr=uint32
  _Feature Switch_ : BusCreator  Inputs=2
  Feature Switch : Outport
  wires:
  _Feature Switch_/1 -> Feature Switch/1  "Feature Switch"
  Const_sigSevereKSIOvervoltage Countdown Start Value/1 -> _Feature Switch_/1  "sigSevereKSIOvervoltage Countdown Start Value"
  Const_sigSevereKSIOvervoltage Feature Switch/1 -> _Feature Switch_/2  "sigSevereKSIOvervoltage Feature Switch"

== system DriveSystemControl/Bus Configuration (1) - In/Manipulation/Virya Controller CAN File 08082024/WIP/CANChannel/PDUs/TCU03/sigSevereKSIOvervoltage/ISignal Overwrite Value ==
  Const_sigSevereKSIOvervoltage Overwrite Value : Constant  Value=0  OutDataTypeStr=uint8
  _ISignal Overwrite Value_ : BusCreator  Inputs=1
  ISignal Overwrite Value : Outport
  wires:
  _ISignal Overwrite Value_/1 -> ISignal Overwrite Value/1  "ISignal Overwrite Value"
  Const_sigSevereKSIOvervoltage Overwrite Value/1 -> _ISignal Overwrite Value_/1  "sigSevereKSIOvervoltage Overwrite Value"

== system DriveSystemControl/Bus Configuration (1) - In/Manipulation/Virya Controller CAN File 08082024/WIP/CANChannel/PDUs/TCU03/sigSevereKSIUndervoltage/Feature Switch ==
  Const_sigSevereKSIUndervoltage Countdown Start Value : Constant  Value=0  OutDataTypeStr=uint32
  Const_sigSevereKSIUndervoltage Feature Switch : Constant  Value=0  OutDataTypeStr=uint32
  _Feature Switch_ : BusCreator  Inputs=2
  Feature Switch : Outport
  wires:
  _Feature Switch_/1 -> Feature Switch/1  "Feature Switch"
  Const_sigSevereKSIUndervoltage Countdown Start Value/1 -> _Feature Switch_/1  "sigSevereKSIUndervoltage Countdown Start Value"
  Const_sigSevereKSIUndervoltage Feature Switch/1 -> _Feature Switch_/2  "sigSevereKSIUndervoltage Feature Switch"

== system DriveSystemControl/Bus Configuration (1) - In/Manipulation/Virya Controller CAN File 08082024/WIP/CANChannel/PDUs/TCU03/sigSevereKSIUndervoltage/ISignal Overwrite Value ==
  Const_sigSevereKSIUndervoltage Overwrite Value : Constant  Value=0  OutDataTypeStr=uint8
  _ISignal Overwrite Value_ : BusCreator  Inputs=1
  ISignal Overwrite Value : Outport
  wires:
  _ISignal Overwrite Value_/1 -> ISignal Overwrite Value/1  "ISignal Overwrite Value"
  Const_sigSevereKSIUndervoltage Overwrite Value/1 -> _ISignal Overwrite Value_/1  "sigSevereKSIUndervoltage Overwrite Value"

== system DriveSystemControl/Bus Configuration (1) - In/Manipulation/Virya Controller CAN File 08082024/WIP/CANChannel/PDUs/TCU03/sigSinCosMisalignment/Feature Switch ==
  Const_sigSinCosMisalignment Countdown Start Value : Constant  Value=0  OutDataTypeStr=uint32
  Const_sigSinCosMisalignment Feature Switch : Constant  Value=0  OutDataTypeStr=uint32
  _Feature Switch_ : BusCreator  Inputs=2
  Feature Switch : Outport
  wires:
  _Feature Switch_/1 -> Feature Switch/1  "Feature Switch"
  Const_sigSinCosMisalignment Countdown Start Value/1 -> _Feature Switch_/1  "sigSinCosMisalignment Countdown Start Value"
  Const_sigSinCosMisalignment Feature Switch/1 -> _Feature Switch_/2  "sigSinCosMisalignment Feature Switch"

== system DriveSystemControl/Bus Configuration (1) - In/Manipulation/Virya Controller CAN File 08082024/WIP/CANChannel/PDUs/TCU03/sigSinCosMisalignment/ISignal Overwrite Value ==
  Const_sigSinCosMisalignment Overwrite Value : Constant  Value=0  OutDataTypeStr=uint8
  _ISignal Overwrite Value_ : BusCreator  Inputs=1
  ISignal Overwrite Value : Outport
  wires:
  _ISignal Overwrite Value_/1 -> ISignal Overwrite Value/1  "ISignal Overwrite Value"
  Const_sigSinCosMisalignment Overwrite Value/1 -> _ISignal Overwrite Value_/1  "sigSinCosMisalignment Overwrite Value"

== system DriveSystemControl/Bus Configuration (1) - In/Manipulation/Virya Controller CAN File 08082024/WIP/CANChannel/PDUs/TCU03/sigSinCosSensorFault/Feature Switch ==
  Const_sigSinCosSensorFault Countdown Start Value : Constant  Value=0  OutDataTypeStr=uint32
  Const_sigSinCosSensorFault Feature Switch : Constant  Value=0  OutDataTypeStr=uint32
  _Feature Switch_ : BusCreator  Inputs=2
  Feature Switch : Outport
  wires:
  _Feature Switch_/1 -> Feature Switch/1  "Feature Switch"
  Const_sigSinCosSensorFault Countdown Start Value/1 -> _Feature Switch_/1  "sigSinCosSensorFault Countdown Start Value"
  Const_sigSinCosSensorFault Feature Switch/1 -> _Feature Switch_/2  "sigSinCosSensorFault Feature Switch"

== system DriveSystemControl/Bus Configuration (1) - In/Manipulation/Virya Controller CAN File 08082024/WIP/CANChannel/PDUs/TCU03/sigSinCosSensorFault/ISignal Overwrite Value ==
  Const_sigSinCosSensorFault Overwrite Value : Constant  Value=0  OutDataTypeStr=uint8
  _ISignal Overwrite Value_ : BusCreator  Inputs=1
  ISignal Overwrite Value : Outport
  wires:
  _ISignal Overwrite Value_/1 -> ISignal Overwrite Value/1  "ISignal Overwrite Value"
  Const_sigSinCosSensorFault Overwrite Value/1 -> _ISignal Overwrite Value_/1  "sigSinCosSensorFault Overwrite Value"

== system DriveSystemControl/Bus Configuration (1) - In/Manipulation/Virya Controller CAN File 08082024/WIP/CANChannel/PDUs/TCU03/sigStallDetected/Feature Switch ==
  Const_sigStallDetected Countdown Start Value : Constant  Value=0  OutDataTypeStr=uint32
  Const_sigStallDetected Feature Switch : Constant  Value=0  OutDataTypeStr=uint32
  _Feature Switch_ : BusCreator  Inputs=2
  Feature Switch : Outport
  wires:
  _Feature Switch_/1 -> Feature Switch/1  "Feature Switch"
  Const_sigStallDetected Countdown Start Value/1 -> _Feature Switch_/1  "sigStallDetected Countdown Start Value"
  Const_sigStallDetected Feature Switch/1 -> _Feature Switch_/2  "sigStallDetected Feature Switch"

== system DriveSystemControl/Bus Configuration (1) - In/Manipulation/Virya Controller CAN File 08082024/WIP/CANChannel/PDUs/TCU03/sigStallDetected/ISignal Overwrite Value ==
  Const_sigStallDetected Overwrite Value : Constant  Value=0  OutDataTypeStr=uint8
  _ISignal Overwrite Value_ : BusCreator  Inputs=1
  ISignal Overwrite Value : Outport
  wires:
  _ISignal Overwrite Value_/1 -> ISignal Overwrite Value/1  "ISignal Overwrite Value"
  Const_sigStallDetected Overwrite Value/1 -> _ISignal Overwrite Value_/1  "sigStallDetected Overwrite Value"
